simulink model "Linearizzato"  (R2020b)
settings: Solver=ode45  StartTime=0.0  StopTime=100  RelTol=1e-6
values from neighbouring files (symbols this model uses):
  A_t = [0 1 0 0 ... (first row only)    [Assignment7Mat.m]
  alpha = 1    [Assignment7Mat.m]
  BP = horzcat(B_t, P_t)    [Assignment7Mat.m]
  C_te = [1 0 0 0]    [Assignment7Mat.m]
  d1_amp = 0.5    [Assignment7Mat.m]
  d1_period = 50    [Assignment7Mat.m]
  K = -ack*pDesA    [Assignment7Mat.m]
  L = Gamma - K*Pi    [Assignment7Mat.m]
  omega = 0.1    [Assignment7Mat.m]
  Q_te = [-1 0 0]    [Assignment7Mat.m]
  x0 = [0 0 0 0]    [Assignment7Mat.m]
settings Model: Creator=Paolo  LastModifiedBy=Paolo

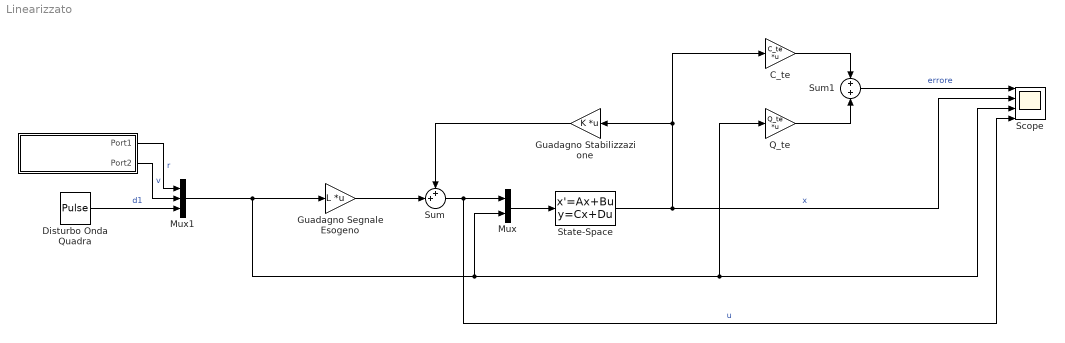
== system Linearizzato ==
  "   " : Subsystem  mask(Differential Equation Editor (DEE)){}
      settings: OpenFcn=diffeqed
      mask Display: disp('Sistema Esogeno')
  C_te : Gain  Gain=C_te  Multiplication=Matrix(K*u)
  Disturbo Onda Quadra : DiscretePulseGenerator  PulseType=Time based  Amplitude=d1_amp  Period=d1_period  PulseWidth=50
  Guadagno Stabilizzazione : Gain  Gain=K  Multiplication=Matrix(K*u)
  Guadagno Segnale Esogeno : Gain  Gain=L  Multiplication=Matrix(K*u)
  Mux : Mux  Inputs=2
  Mux1 : Mux  Inputs=3
  Q_te : Gain  Gain=Q_te  Multiplication=Matrix(K*u)
  Scope : Scope  NumInputPorts=4
  State-Space : StateSpace  A=A_t  B=BP  C=[1 0 0 0; 0 1 0 0; 0 0 1 0; 0 0 0 1]  D=[0 0 0 0; 0 0 0 0; 0 0 0 0; 0 0 0 0]  InitialCondition=x0
  Sum : Sum  Inputs=++|
  Sum1 : Sum  Inputs=+|+
  wires:
  "   "/1(Port1) -> Mux1/1  "r"
  Disturbo Onda Quadra/1 -> Mux1/3  "d1"
  "   "/2(Port2) -> Mux1/2  "v"
  Mux1/1 -> Mux/2, Scope/3, Q_te/1, Guadagno Segnale Esogeno/1
  Guadagno Segnale Esogeno/1 -> Sum/2
  Sum/1 -> Scope/4, Mux/1  "u"
  Mux/1 -> State-Space/1
  State-Space/1 -> C_te/1, Guadagno Stabilizzazione/1, Scope/2  "x"
  Guadagno Stabilizzazione/1 -> Sum/1
  C_te/1 -> Sum1/1
  Q_te/1 -> Sum1/2
  Sum1/1 -> Scope/1  "errore"

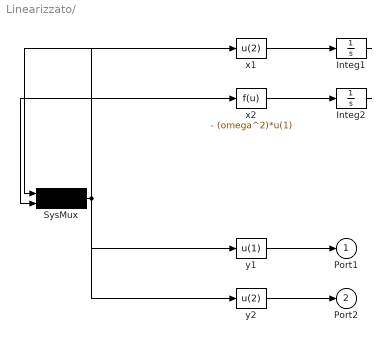
== system Linearizzato/    ==
  Integ1 : Integrator
  Integ2 : Integrator  InitialCondition=omega*alpha
  SysMux : Mux  Inputs=2
  x1 : Fcn  Expr=u(2)
  x2 : Fcn  Expr=- (omega^2)*u(1)
  y1 : Fcn  Expr=u(1)
  y2 : Fcn  Expr=u(2)
  Port1 : Outport
  Port2 : Outport  Port=2
  wires:
  SysMux/1 -> x1/1, x2/1, y1/1, y2/1
  x1/1 -> Integ1/1
  Integ1/1 -> SysMux/1
  x2/1 -> Integ2/1
  Integ2/1 -> SysMux/2
  y1/1 -> Port1/1
  y2/1 -> Port2/1
